simulink model "Blinker_31_exp"  (R2021b)
settings: Solver=FixedStepDiscrete  StartTime=0.0  StopTime=10.0  FixedStep=Ts  RelTol=1e-3  EnableMultiTasking=on
PreLoadFcn:
  | Ts = 0.05;
  | Ts_1 = 0.05;   % for runnable blink_signal
  | Ts_2 = 1;       % for runnable validate_ignition
  | 
  | SetEnumTypeBlink;
libraries: simulink x1
settings Model: Creator=urempel  LastModifiedBy=adish
settings SolverCC: AlgebraicLoopSolver=TrustRegion
settings DataIOCC: LimitDataPoints=on  SaveFormat=Array  ReturnWorkspaceOutputs=off
settings OptimizationCC: LifeSpan=1  EfficientTunableParamExpr=on
settings DebuggingCC: SolverPrmCheckMsg=warning  AllowSymbolicDim=off  SFUnexpectedBacktrackingDiag=warning  SFNoUnconditionalDefaultTransitionDiag=warning  SFExecutionAtInitializationDiag=none  SFMachineParentedDataDiag=warning  ArithmeticOperatorsInVariantConditions=warning
settings ModelReferenceCC: PropagateSignalLabelsOutOfModel=off
settings SFSimCC: SimUseLocalCustomCode=off  SimGenImportedTypeDefs=on  MATLABDynamicMemAlloc=off  CustomCodeUndefinedFunction=UseInterfaceOnly
settings RTWCC: Description=Embedded Coder  SystemTargetFile=ert.tlc  GenCodeOnly=on  TemplateMakefile=ert_default_tmf  RTWUseLocalCustomCode=off  IncludeHyperlinkInReport=on
settings CodeAppCC: IgnoreCustomStorageClasses=off  StateflowObjectComments=on
settings ERTTargetCC: MultiwordLength=2048  GenerateSampleERTMain=on  ERTCustomFileTemplate=example_file_process.tlc  ConvertIfToSwitch=off  SuppressUnreachableDefaultCases=off
settings ConfigComp: CovMetricSettings=dw  CovSaveCumulativeToWorkspaceVar=on  CovSaveSingleToWorkspaceVar=on  CovExternalEMLEnable=off  CovSFcnEnable=off

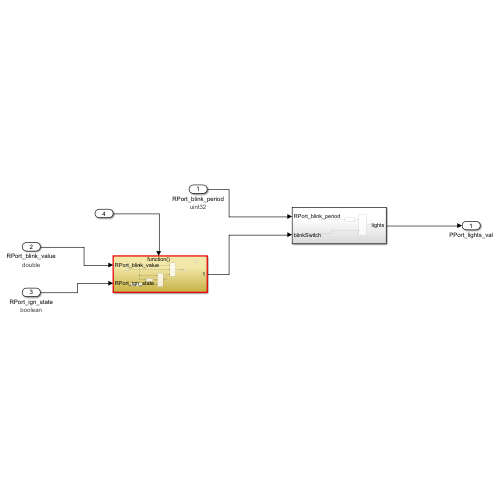
[thumbnail: Simulink's stored preview of the top-level diagram]
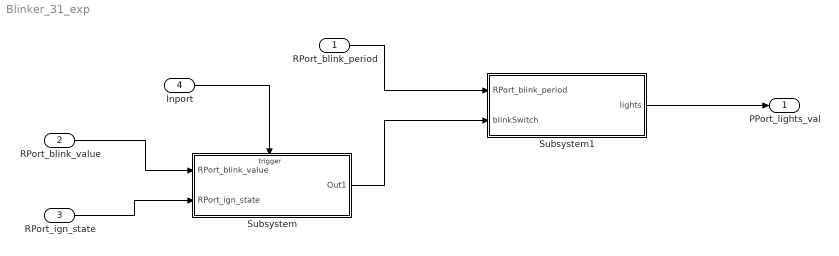
== system Blinker_31_exp ==
  RPort_blink_period : Inport  OutDataTypeStr=uint32
      settings: AttributesFormatString=%<OutDataTypeStr>
  RPort_blink_value : Inport  Port=2  OutDataTypeStr=double
      settings: AttributesFormatString=%<OutDataTypeStr>
  RPort_ign_state : Inport  Port=3  OutDataTypeStr=boolean
      settings: AttributesFormatString=%<OutDataTypeStr>
  Inport : Inport  Port=4  SampleTime=Ts_1  OutputFunctionCall=on
  Subsystem : Subsystem
  Subsystem1 : Subsystem
  PPort_lights_val : Outport  InitialOutput=0
  wires:
  RPort_blink_value/1 -> Subsystem/1(RPort_blink_value)
  RPort_ign_state/1 -> Subsystem/2(RPort_ign_state)
  RPort_blink_period/1 -> Subsystem1/1(RPort_blink_period)
  Subsystem/1(Out1) -> Subsystem1/2(blinkSwitch)
  Subsystem1/1(lights) -> PPort_lights_val/1
  Inport/1 -> Subsystem/Trigger

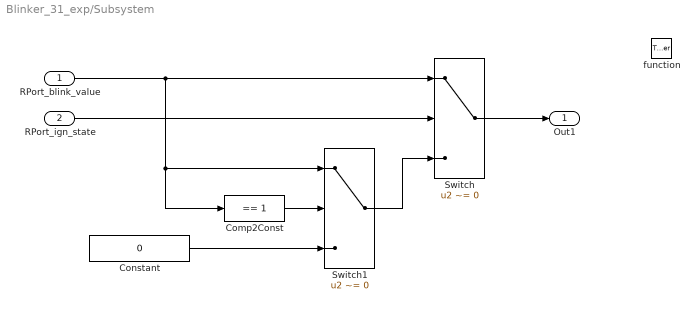
== system Blinker_31_exp/Subsystem ==
  RPort_blink_value : Inport  OutDataTypeStr=double
      settings: AttributesFormatString=%<OutDataTypeStr>
  RPort_ign_state : Inport  Port=2  OutDataTypeStr=boolean
      settings: AttributesFormatString=%<OutDataTypeStr>
  function : TriggerPort  TriggerType=function-call  VariantControl=(inherit)  PropagateVarSize=Only when enabling  SampleTimeType=periodic  SampleTime=-1  PortDimensions=1
  Comp2Const : simulink/Logic and Bit Operations/Compare To Constant  relop===  const=1  OutDataTypeStr=boolean
  Constant : Constant  Value=0
      settings: AttributesFormatString=%<OutDataTypeStr>
  Switch : Switch  Criteria=u2 ~= 0
  Switch1 : Switch  Criteria=u2 ~= 0
  Out1 : Outport
  wires:
  Constant/1 -> Switch1/3
  Comp2Const/1 -> Switch1/2
  RPort_blink_value/1 -> Switch1/1, Comp2Const/1, Switch/1
  Switch1/1 -> Switch/3
  RPort_ign_state/1 -> Switch/2
  Switch/1 -> Out1/1

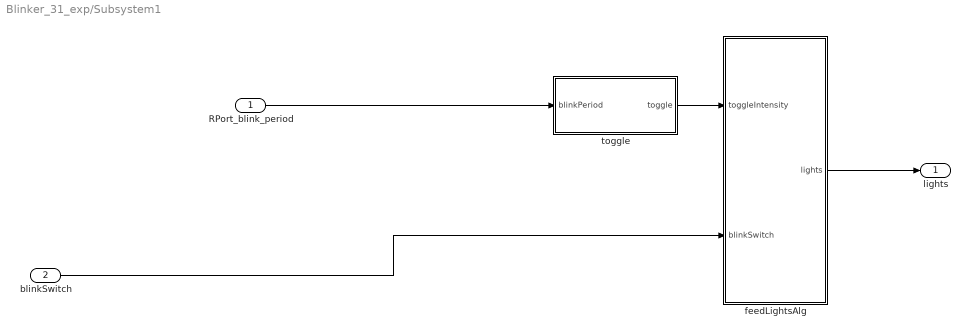
== system Blinker_31_exp/Subsystem1 ==
  RPort_blink_period : Inport  OutDataTypeStr=uint32
      settings: AttributesFormatString=%<OutDataTypeStr>
  blinkSwitch : Inport  Port=2
  feedLightsAlg : MATLAB Function  TreatAsAtomicUnit=on
  toggle : Stateflow chart  TreatAsAtomicUnit=on
  lights : Outport
  wires:
  toggle/1(toggle) -> feedLightsAlg/1(toggleIntensity)
  RPort_blink_period/1 -> toggle/1(blinkPeriod)
  feedLightsAlg/1(lights) -> lights/1
  blinkSwitch/1 -> feedLightsAlg/2(blinkSwitch)

== matlab function Blinker_31_exp/Subsystem1/feedLightsAlg ==
  data: toggleIntensity input boolean; blinkSwitch input double; lights output boolean size=[1,2]
function lights = feedLightsAlg(toggleIntensity, blinkSwitch )
%#codegen
switch blinkSwitch
	case BlinkerValues.right
		lights = [false, toggleIntensity];
	case BlinkerValues.left
		lights = [toggleIntensity, false];
	case BlinkerValues.hazard
		lights = [toggleIntensity, toggleIntensity];
	otherwise
		lights = [false, false];
end

== stateflow chart Blinker_31_exp/Subsystem1/toggle ==
  (default) -> (junction 2)
  (junction 2) -> (junction 7) [order 1] : [blinkPeriod <= cntr]
  (junction 2) -> (junction 3) [order 2] : {
      | cntr++;
      | }
  (junction 7) -> (junction 8) : {
      | toggle = !toggle;
      | cntr = 1;
      | }
  (junction 8) -> (junction 3)
  data: toggle output boolean =0; blinkPeriod input uint32; cntr local uint32 =0
